simulink model "gamepadcontroller"  (R2024b)
settings: Solver=VariableStepAuto  StartTime=0.0  StopTime=100.0  RelTol=1e-3
undefined symbols (not defined in the file): f, LF
libraries: instrumentseriallib x2, vrlib x1, instrumentlib x1
settings Model: Creator=PC  LastModifiedBy=PC

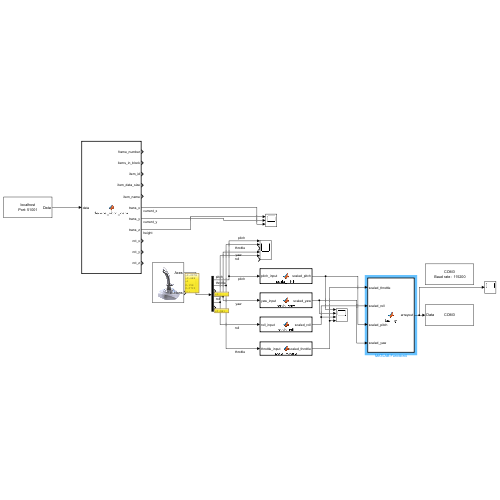
[thumbnail: Simulink's stored preview of the top-level diagram]
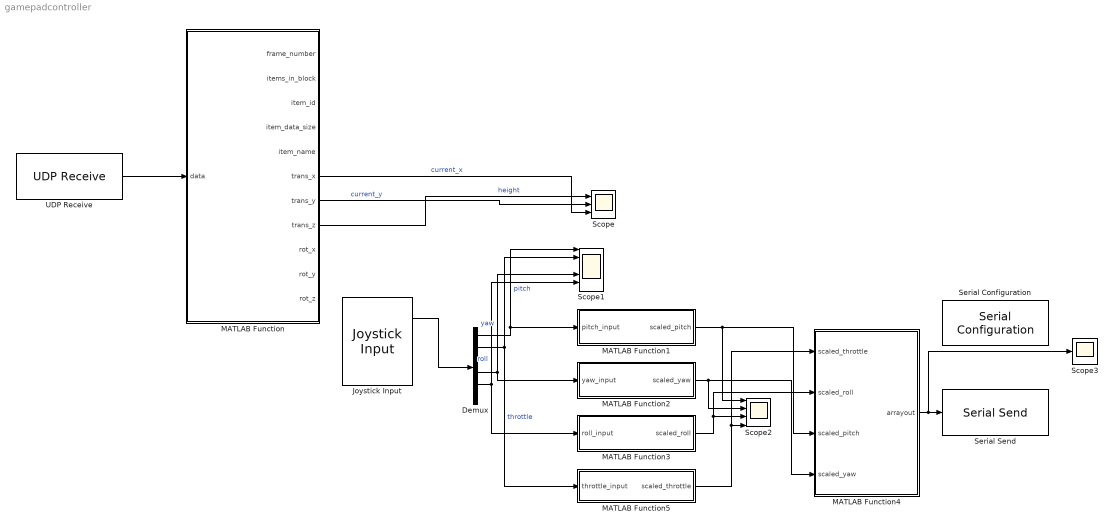
== system gamepadcontroller ==
  Demux : Demux  Outputs=6
  Joystick Input : vrlib/Joystick Input  joyid=1  adjustports=on  forcefeed=off
  MATLAB Function : MATLAB Function  TreatAsAtomicUnit=on
  MATLAB Function1 : MATLAB Function  TreatAsAtomicUnit=on
  MATLAB Function2 : MATLAB Function  TreatAsAtomicUnit=on
  MATLAB Function3 : MATLAB Function  TreatAsAtomicUnit=on
  MATLAB Function4 : MATLAB Function  TreatAsAtomicUnit=on
  MATLAB Function5 : MATLAB Function  TreatAsAtomicUnit=on
  Scope : Scope  NumInputPorts=3
  Scope1 : Scope  NumInputPorts=6
  Scope2 : Scope  NumInputPorts=4
  Scope3 : Scope
  Serial Configuration : instrumentseriallib/Serial Configuration  Priority=-200000  PortSel=COM3  Port=COM3  ComPort=COM3  BaudRate=115200  DataBits=8  Parity=none  StopBits=1  ByteOrder=little-endian  FlowControl=none  Timeout=10  SimulateUsing=Interpreted execution  BlockInModel=on  aMode=1
  Serial Send : instrumentseriallib/Serial Send  Priority=1  PortSel=COM3  Port=COM3  ComPort=COM3  Header=[]  Terminator=LF ('\n')  CustomTerminator=[]  EnableBlockingMode=on  SimulateUsing=Interpreted execution  BlockInModel=on  aMode=1
  UDP Receive : instrumentlib/UDP Receive  LocalAddress=localhost  LocalPort=51001  EnablePortSharing=off  Host=localhost  Port=9090  GetLatestData=on  DataSize=[1024, 1]  DataType=uint8  ASCIIFormatting=%f,  Terminator=LF  CustomTerminator=10  ByteOrder=big-endian  EnableBlockingMode=on  Timeout=10  SampleTime=0.02  SimulateUsing=Interpreted execution
  wires:
  UDP Receive/1 -> MATLAB Function/1(data)
  MATLAB Function/8(trans_z) -> Scope/1  "height"
  MATLAB Function/7(trans_y) -> Scope/2  "current_y"
  MATLAB Function/6(trans_x) -> Scope/3  "current_x"
  Joystick Input/1 -> Demux/1
  Demux/1 -> Scope1/1, MATLAB Function1/1(pitch_input)  "pitch"
  Demux/2 -> MATLAB Function5/1(throttle_input), Scope1/2  "throttle"
  Demux/4 -> MATLAB Function2/1(yaw_input), Scope1/4  "yaw"
  Demux/5 -> MATLAB Function3/1(roll_input), Scope1/5  "roll"
  MATLAB Function1/1(scaled_pitch) -> MATLAB Function4/3(scaled_pitch), Scope2/1
  MATLAB Function2/1(scaled_yaw) -> Scope2/2, MATLAB Function4/4(scaled_yaw)
  MATLAB Function3/1(scaled_roll) -> MATLAB Function4/2(scaled_roll), Scope2/3
  MATLAB Function5/1(scaled_throttle) -> MATLAB Function4/1(scaled_throttle), Scope2/4
  MATLAB Function4/1(arrayout) -> Serial Send/1, Scope3/1

== matlab function gamepadcontroller/MATLAB Function1 ==
  data: pitch_input input; scaled_pitch output
function scaled_pitch = scale_pitch(pitch_input)
    % Define the original and target ranges
    a = -0.700;
    b = 0.800;
    c = 500;
    d = 1500;

    % Apply the scaling formula
    scaled_pitch = c + ((pitch_input - a) * (d - c)) / (b - a);
end

== matlab function gamepadcontroller/MATLAB Function ==
  data: data input; frame_number output; items_in_block output; item_id output; item_data_size output; item_name output; trans_x output; trans_y output; trans_z output; rot_x output; rot_y output; rot_z output
function [frame_number, items_in_block, item_id, item_data_size, item_name, ...
    trans_x, trans_y, trans_z, rot_x, rot_y, rot_z] = decode_vicon_data(data)
    % Define expected output sizes explicitly
    % Set up each output as an array with dimensions (1x1) or (8x1) as needed.

    % Initialize output arrays
    frame_number = zeros(1, 1, 'uint32');  % Explicitly scalar output
    items_in_block = zeros(1, 1, 'uint8');  % Explicitly scalar output
    item_id = zeros(1, 1, 'uint8');        % Explicitly scalar output
    item_data_size = zeros(1, 1, 'uint16'); % Explicitly scalar output
    item_name = zeros(24, 1, 'uint8');     % 24 bytes for item name, uint8 array
    trans_x = zeros(1, 1, 'double');       % Scalar, double
    trans_y = zeros(1, 1, 'double');       % Scalar, double
    trans_z = zeros(1, 1, 'double');       % Scalar, double
    rot_x = zeros(1, 1, 'double');         % Scalar, double
    rot_y = zeros(1, 1, 'double');         % Scalar, double
    rot_z = zeros(1, 1, 'double');         % Scalar, double

    % Frame Number (4 bytes, uint32), scalar
    frame_number = typecast(data(1:4), 'uint32');
    
    % ItemsInBlock (1 byte, uint8)
    items_in_block = uint8(data(5));  % Scalar uint8
    
    % Item ID (1 byte, uint8) (0 for object data)
    item_id = uint8(data(6));  % Scalar uint8
    
    % Item Data Size (2 bytes, uint16)
    item_data_size = typecast(data(7:8), 'uint16');  % Scalar uint16
    
    % Item Name (24 bytes, uint8) converted from char
    item_name = uint8(data(9:32));  % Cast to uint8 (ASCII values of characters)
    
    % Translation (TransX, TransY, TransZ) - 8 bytes each (double)
    trans_x = typecast(data(33:40), 'double');
    trans_y = typecast(data(41:48), 'double');
    trans_z = typecast(data(49:56), 'double');
    
    % Rotation (RotX, RotY, RotZ) - 8 bytes each (double)
    rot_x = typecast(data(57:64), 'double');
    rot_y = typecast(data(65:72), 'double');
    rot_z = typecast(data(73:80), 'double');
end

== matlab function gamepadcontroller/MATLAB Function2 ==
  data: yaw_input input; scaled_yaw output
function scaled_yaw = scale_yaw(yaw_input)
    % Define the original and target ranges
    a = -0.695;
    b = 0.980;
    c = 500;
    d = 1500;

    % Apply the scaling formula
    scaled_yaw = c + ((yaw_input - a) * (d - c)) / (b - a);
end

== matlab function gamepadcontroller/MATLAB Function3 ==
  data: roll_input input; scaled_roll output
function scaled_roll = scale_roll(roll_input)
    % Define the original and target ranges
    a = -0.867;
    b = 0.873;
    c = 500;
    d = 1500;

    % Apply the scaling formula
    scaled_roll = c + ((roll_input - a) * (d - c)) / (b - a);
end

== matlab function gamepadcontroller/MATLAB Function4 ==
  data: scaled_throttle input; scaled_roll input; arrayout output; scaled_pitch input; scaled_yaw input
% MATLAB Function code
function arrayout = toarray(scaled_throttle, scaled_roll, scaled_pitch, scaled_yaw)
    % Cast each input value to int32
    desiredthrottle = int16(scaled_throttle)
    desiredroll = int16(scaled_roll);  
    desiredpitch = int16(scaled_pitch);  
    desiredyaw = int16(scaled_yaw);  
    
    % Store the values in an array
    arrayout = [desiredthrottle, desiredroll, desiredpitch, desiredyaw];
    
    % Print the values as comma-separated integers with newline
    fprintf('%d,%d,%d,%d\n', arrayout(1), arrayout(2), arrayout(3), arrayout(4));
end

== matlab function gamepadcontroller/MATLAB Function5 ==
  data: throttle_input input; scaled_throttle output
function scaled_throttle = scale_throttle(throttle_input)
    % Define the original and target ranges
    a = -0.6875;
    b = 0.840;
    c = 500;
    d = 1500;

    % Apply the scaling formula
    scaled_throttle = c + ((throttle_input - a) * (d - c)) / (b - a);
end
